simulink model "ex1s"  (R2013a)
settings: Solver=ode45  StartTime=0.0  StopTime=10.0  RelTol=1e-3
settings Model: Creator=Edward  LastModifiedBy=Edward

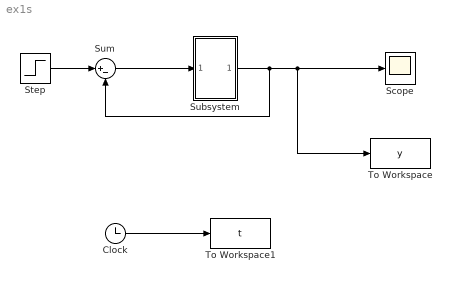
== system ex1s ==
  Clock : Clock
  Scope : Scope
  Step : Step  SampleTime=0
  Subsystem : Subsystem  mask{a=10, b=0.6}
      mask prompts: a "val a"; b "val b"
      mask Callback a:
      | if str2num(get_param(gcb,'a'))<0
      |     error('negativa!!!')
      | end
      mask Callback b:
      | if str2num(get_param(gcb,'b'))<0
      |     error('negativa!!!')
      | end
  Sum : Sum  Inputs=|+-
  To Workspace : ToWorkspace  VariableName=y  SampleTime=-1
  To Workspace1 : ToWorkspace  VariableName=t  SampleTime=-1
  wires:
  Step/1 -> Sum/1
  Sum/1 -> Subsystem/1(In1)
  Subsystem/1(Out1) -> To Workspace/1, Scope/1, Sum/2
  Clock/1 -> To Workspace1/1

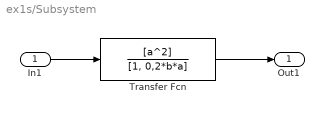
== system ex1s/Subsystem ==
  In1 : Inport
  Transfer Fcn : TransferFcn  Numerator=[a^2]  Denominator=[1, 0,2*b*a]
  Out1 : Outport
  wires:
  Transfer Fcn/1 -> Out1/1
  In1/1 -> Transfer Fcn/1
